simulink model "tutorial27_msd_models"  (R2025a)
settings: Solver=VariableStepAuto  StartTime=0.0  StopTime=10.0  RelTol=1e-3
settings Model: Creator=xing2  LastModifiedBy=xing2

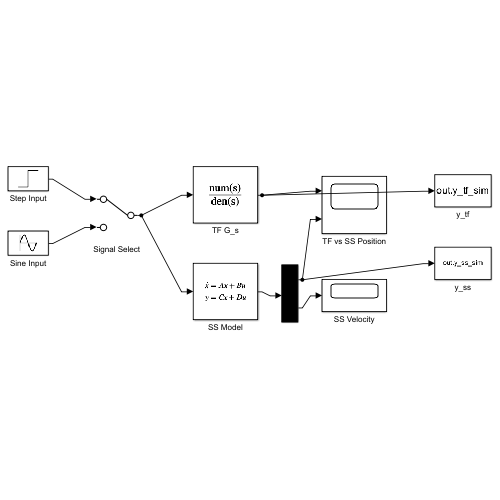
[thumbnail: Simulink's stored preview of the top-level diagram]
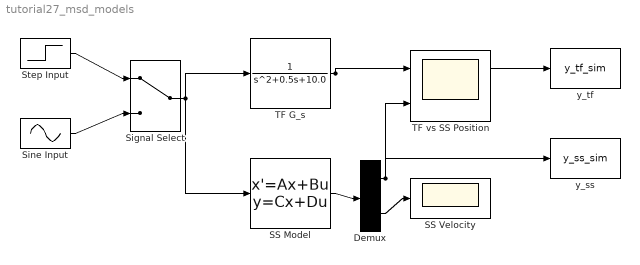
== system tutorial27_msd_models ==
  Demux : Demux  Outputs=2
  SS Model : StateSpace  A=[0 1;-10.0000 -0.5000]  B=[0;1]  C=eye(2)  D=[0;0]  InitialCondition=[0;0]
  SS Velocity : Scope
  Signal Select : ManualSwitch
  Sine Input : Sin  Frequency=3.1623  SampleTime=0
  Step Input : Step  Time=0.5  SampleTime=0
  TF G_s : TransferFcn  Denominator=[1.0 0.5 10.0]
  TF vs SS Position : Scope  NumInputPorts=2
  y_ss : ToWorkspace  VariableName=y_ss_sim  SaveFormat=Timeseries  SampleTime=-1
  y_tf : ToWorkspace  VariableName=y_tf_sim  SaveFormat=Timeseries  SampleTime=-1
  wires:
  Step Input/1 -> Signal Select/1
  Sine Input/1 -> Signal Select/2
  Signal Select/1 -> TF G_s/1, SS Model/1
  SS Model/1 -> Demux/1
  TF G_s/1 -> TF vs SS Position/1, y_tf/1
  Demux/1 -> TF vs SS Position/2, y_ss/1
  Demux/2 -> SS Velocity/1
